simulink model "two_chamber_membrane"  (R2025a)
settings: Solver=VariableStepAuto  StartTime=0.0  StopTime=1000000  RelTol=1e-3  AbsTol=1e-3
libraries: nesl_utility x1
settings Model: Creator=degoede  LastModifiedBy=degoede
settings SolverCC: AutoScaleAbsTol=off
settings SimscapeCC: SimscapeLogType=all  SimscapeLogSimulationStatistics=on  SimscapeLogOpenViewer=on

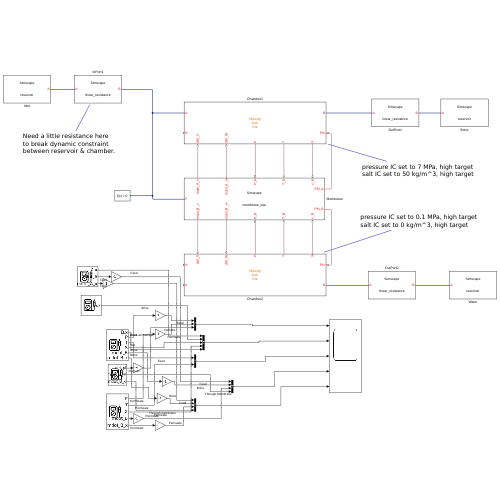
[thumbnail: Simulink's stored preview of the top-level diagram]
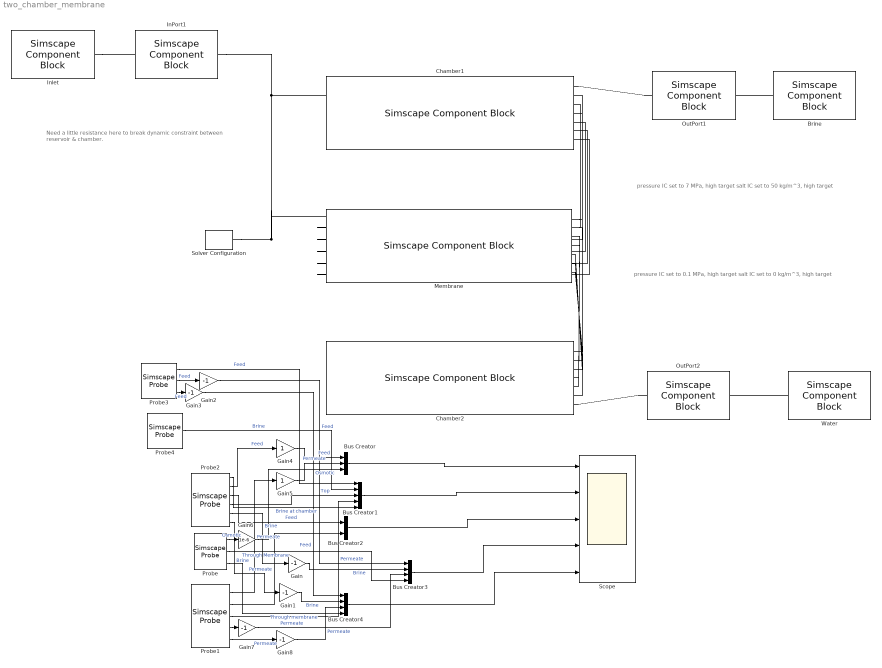
== system two_chamber_membrane ==
  note: pressure IC set to 7 MPa, high target
      | salt IC set to 50 kg/m^3, high target
  note: Need a little resistance here
      | to break dynamic constraint
      | between reservoir & chamber.
  note: pressure IC set to 0.1 MPa, high target
      | salt IC set to 0 kg/m^3, high target
  Brine : SimscapeComponentBlock  SourceFile=customization.solution.elements.reservoir  ComponentPath=customization.solution.elements.reservoir  ComponentVariants="[\"customization.solution.elements.reservoir\"]"  ComponentVariantNames="[\"reservoir\"]"  ClassName=reservoir  SchemaVersion=1  pressure_spec=foundation.enum.pressure_spec.atmospheric  reservoir_pressure=0.101325 MPa  reservoir_temperature=293.15 K  reservoir_concentration=50 kg/m^3  area=1 cm^2
      settings: CopyFcn=simscape.sscblock.internal.componentBlockCallback(gcbh,'COPY')  PreCopyFcn=simscape.sscblock.internal.componentBlockCallback(gcbh,'PRECOPY')  PreDeleteFcn=simscape.sscblock.internal.componentBlockCallback(gcbh,'PREDELETE')  InternalSimscapePortConfiguration="{\"Bottom\":[],\"Left\":[{\"id\":\"A\",\"label\":\"A\",\"type\":\"customization.solution.solution\"}],\"Right\":[],\"Top\":[]}"
      mask Type: Reservoir (SS)
  Bus Creator : BusCreator  Inputs=3
  Bus Creator1 : BusCreator  Inputs=5
  Bus Creator2 : BusCreator  Inputs=2
  Bus Creator3 : BusCreator  Inputs=4
  Bus Creator4 : BusCreator  Inputs=4
  Chamber1 : SimscapeComponentBlock  SourceFile=customization.solution.elements.constant_volume_chamber  ComponentPath=customization.solution.elements.constant_volume_chamber  ComponentVariants="[\"customization.solution.elements.constant_volume_chamber\"]"  ComponentVariantNames="[\"constant_volume_chamber\"]"  ClassName=constant_volume_chamber  SchemaVersion=1  volume=0.001 m^3  num_ports=foundation.enum.num_ports.two  area_A=1 cm^2  area_B=1 cm^2  area_C=0.01 m^2  area_D=0.01 m^2  m_measure=false  p_measure=true  t_measure=true  x_measure=true  p_I_specify=on  p_I_priority=High  p_I=7 MPa  p_I_nominal_specify=off  p_I_nominal_value=1  p_I_nominal_unit=MPa  T_I_specify=off  T_I_priority=High  T_I=293.15 K  T_I_nominal_specify=off  T_I_nominal_value=1  T_I_nominal_unit=K  u_I_specify=off  u_I_priority=None  u_I=83.906 kJ/kg  u_I_nominal_specify=off  u_I_nominal_value=1  u_I_nominal_unit=kJ/kg  rho_I_specify=off  rho_I_priority=None  rho_I=998.21 kg/m^3  rho_I_nominal_specify=off  rho_I_nominal_value=1  rho_I_nominal_unit=kg/m^3  x_I_specify=on  x_I_priority=High  x_I=50 kg/m^3  x_I_nominal_specify=off  x_I_nominal_value=1  x_I_nominal_unit=kg/m^3
      settings: CopyFcn=simscape.sscblock.internal.componentBlockCallback(gcbh,'COPY')  PreCopyFcn=simscape.sscblock.internal.componentBlockCallback(gcbh,'PRECOPY')  PreDeleteFcn=simscape.sscblock.internal.componentBlockCallback(gcbh,'PREDELETE')  InternalSimscapePortConfiguration="{\"Bottom\":[{\"id\":\"dM_X\",\"label\":\"dM_X\",\"type\":\"input\"},{\"id\":\"dM_W\",\"label\":\"dM_W\",\"type\":\"input\"},{\"id\":\"P\",\"label\":\"P\",\"type\":\"output\"},{\"id\":\"T\",\"label\":\"T\",\"type\":\"output\"},{\"id\":\"X\",\"label\":\"X\",\"type\":\"output\"}],\"Left\":[{\"id\":\"A\",\"label\":\"A\",\"type\":\"customization.solution.solution\"},{\"id\":\"H\",\"label\":\"H\",\"type\":\"foundation.thermal.thermal\"}],\"Right\":[{\"id\":\"B\",\"label\":\"B\",\"type\":\"customization.solution.solution\"},{\"id\":\"Phi\",\"label\":\"Phi\",\"type\":\"input\"}],\"Top\":[]}"
      mask Type: Constant Volume Chamber (SS)
  Chamber2 : SimscapeComponentBlock  SourceFile=customization.solution.elements.constant_volume_chamber  ComponentPath=customization.solution.elements.constant_volume_chamber  ComponentVariants="[\"customization.solution.elements.constant_volume_chamber\"]"  ComponentVariantNames="[\"constant_volume_chamber\"]"  ClassName=constant_volume_chamber  SchemaVersion=1  volume=0.001 m^3  num_ports=foundation.enum.num_ports.two  area_A=1 cm^2  area_B=1 cm^2  area_C=0.01 m^2  area_D=0.01 m^2  m_measure=false  p_measure=true  t_measure=true  x_measure=true  p_I_specify=on  p_I_priority=High  p_I=0.1 MPa  p_I_nominal_specify=off  p_I_nominal_value=1  p_I_nominal_unit=MPa  T_I_specify=off  T_I_priority=High  T_I=293.15 K  T_I_nominal_specify=off  T_I_nominal_value=1  T_I_nominal_unit=K  u_I_specify=off  u_I_priority=None  u_I=83.906 kJ/kg  u_I_nominal_specify=off  u_I_nominal_value=1  u_I_nominal_unit=kJ/kg  rho_I_specify=off  rho_I_priority=None  rho_I=998.21 kg/m^3  rho_I_nominal_specify=off  rho_I_nominal_value=1  rho_I_nominal_unit=kg/m^3  x_I_specify=on  x_I_priority=High  x_I=0 kg/m^3  x_I_nominal_specify=off  x_I_nominal_value=1  x_I_nominal_unit=kg/m^3
      settings: CopyFcn=simscape.sscblock.internal.componentBlockCallback(gcbh,'COPY')  PreCopyFcn=simscape.sscblock.internal.componentBlockCallback(gcbh,'PRECOPY')  PreDeleteFcn=simscape.sscblock.internal.componentBlockCallback(gcbh,'PREDELETE')  InternalSimscapePortConfiguration="{\"Bottom\":[{\"id\":\"dM_X\",\"label\":\"dM_X\",\"type\":\"input\"},{\"id\":\"dM_W\",\"label\":\"dM_W\",\"type\":\"input\"},{\"id\":\"P\",\"label\":\"P\",\"type\":\"output\"},{\"id\":\"T\",\"label\":\"T\",\"type\":\"output\"},{\"id\":\"X\",\"label\":\"X\",\"type\":\"output\"}],\"Left\":[{\"id\":\"A\",\"label\":\"A\",\"type\":\"customization.solution.solution\"},{\"id\":\"H\",\"label\":\"H\",\"type\":\"foundation.thermal.thermal\"}],\"Right\":[{\"id\":\"B\",\"label\":\"B\",\"type\":\"customization.solution.solution\"},{\"id\":\"Phi\",\"label\":\"Phi\",\"type\":\"input\"}],\"Top\":[]}"
      mask Type: Constant Volume Chamber (SS)
  Gain{,1..3,7..8} (6 alike) : Gain  Gain=-1
  Gain4 : Gain
  Gain5 : Gain
  Gain6 : Gain  Gain=1e-6
  InPort1 : SimscapeComponentBlock  SourceFile=customization.solution.elements.linear_resistance  ComponentPath=customization.solution.elements.linear_resistance  ComponentVariants="[\"customization.solution.elements.linear_resistance\"]"  ComponentVariantNames="[\"linear_resistance\"]"  ClassName=linear_resistance  SchemaVersion=1  R=64.23e3 Pa*s/m^3  area=1 cm^2
      settings: CopyFcn=simscape.sscblock.internal.componentBlockCallback(gcbh,'COPY')  PreCopyFcn=simscape.sscblock.internal.componentBlockCallback(gcbh,'PRECOPY')  PreDeleteFcn=simscape.sscblock.internal.componentBlockCallback(gcbh,'PREDELETE')  InternalSimscapePortConfiguration="{\"Bottom\":[],\"Left\":[{\"id\":\"A\",\"label\":\"A\",\"type\":\"customization.solution.solution\"}],\"Right\":[{\"id\":\"B\",\"label\":\"B\",\"type\":\"customization.solution.solution\"}],\"Top\":[]}"
      mask Type: Linear Resistance (SS)
  Inlet : SimscapeComponentBlock  SourceFile=customization.solution.elements.reservoir  ComponentPath=customization.solution.elements.reservoir  ComponentVariants="[\"customization.solution.elements.reservoir\"]"  ComponentVariantNames="[\"reservoir\"]"  ClassName=reservoir  SchemaVersion=1  pressure_spec=foundation.enum.pressure_spec.specified  reservoir_pressure=7 MPa  reservoir_temperature=293.15 K  reservoir_concentration=50 kg/m^3  area=1 cm^2
      settings: CopyFcn=simscape.sscblock.internal.componentBlockCallback(gcbh,'COPY')  PreCopyFcn=simscape.sscblock.internal.componentBlockCallback(gcbh,'PRECOPY')  PreDeleteFcn=simscape.sscblock.internal.componentBlockCallback(gcbh,'PREDELETE')  InternalSimscapePortConfiguration="{\"Bottom\":[],\"Left\":[{\"id\":\"A\",\"label\":\"A\",\"type\":\"customization.solution.solution\"}],\"Right\":[],\"Top\":[]}"
      mask Type: Reservoir (SS)
  Membrane : SimscapeComponentBlock  SourceFile=customization.solution.elements.membrane_eqs  ComponentPath=customization.solution.elements.membrane_eqs  ComponentVariants="[\"customization.solution.elements.membrane_eqs\"]"  ComponentVariantNames="[\"membrane_eqs\"]"  ClassName=membrane_eqs  SchemaVersion=1  A_w=2.57e-12 m^3/(N*s)  B_s=2.30e-8 m/s  A_m=35 m^2
      settings: CopyFcn=simscape.sscblock.internal.componentBlockCallback(gcbh,'COPY')  PreCopyFcn=simscape.sscblock.internal.componentBlockCallback(gcbh,'PRECOPY')  PreDeleteFcn=simscape.sscblock.internal.componentBlockCallback(gcbh,'PREDELETE')  InternalSimscapePortConfiguration="{\"Bottom\":[{\"id\":\"mdot_B_x\",\"label\":\"mdot_B_x\",\"type\":\"output\"},{\"id\":\"mdot_B_w\",\"label\":\"mdot_B_w\",\"type\":\"output\"},{\"id\":\"P_B\",\"label\":\"P_B\",\"type\":\"input\"},{\"id\":\"T_B\",\"label\":\"T_B\",\"type\":\"input\"},{\"id\":\"x_B\",\"label\":\"x_B\",\"type\":\"input\"}],\"Left\":[{\"id\":\"F\",\"label\":\"F\",\"type\":\"customization.solution.solution\"}],\"Right\":[{\"id\":\"Phi_A\",\"label\":\"Phi_A\",\"type\":\"output\"},{\"id\":\"Phi_B\",\"label\":\"Phi_B\",\"type\":\"output\"}],\"Top\":[{\"id\":\"mdot_A_x\",\"label\":\"mdot_A_x\",\"type\":\"output\"},{\"id\":\"mdot_A_w\",\"label\":\"mdot_A_w\",\"type\":\"output\"},{\"id\":\"P_A\",\"label\":\"P_A\",\"type\":\"input\"},{\"id\":\"T_A\",\"label\":\"T_A\",\"type\":\"input\"},{\"id\":\"x_A\",\"label\":\"x_A\",\"type\":\"input\"}]}"
      mask Type: Membrane EQs
  OutPort1 : SimscapeComponentBlock  SourceFile=customization.solution.elements.linear_resistance  ComponentPath=customization.solution.elements.linear_resistance  ComponentVariants="[\"customization.solution.elements.linear_resistance\"]"  ComponentVariantNames="[\"linear_resistance\"]"  ClassName=linear_resistance  SchemaVersion=1  R=64.23e6 Pa*s/m^3  area=1 cm^2
      settings: CopyFcn=simscape.sscblock.internal.componentBlockCallback(gcbh,'COPY')  PreCopyFcn=simscape.sscblock.internal.componentBlockCallback(gcbh,'PRECOPY')  PreDeleteFcn=simscape.sscblock.internal.componentBlockCallback(gcbh,'PREDELETE')  InternalSimscapePortConfiguration="{\"Bottom\":[],\"Left\":[{\"id\":\"A\",\"label\":\"A\",\"type\":\"customization.solution.solution\"}],\"Right\":[{\"id\":\"B\",\"label\":\"B\",\"type\":\"customization.solution.solution\"}],\"Top\":[]}"
      mask Type: Linear Resistance (SS)
  OutPort2 : SimscapeComponentBlock  SourceFile=customization.solution.elements.linear_resistance  ComponentPath=customization.solution.elements.linear_resistance  ComponentVariants="[\"customization.solution.elements.linear_resistance\"]"  ComponentVariantNames="[\"linear_resistance\"]"  ClassName=linear_resistance  SchemaVersion=1  R=64.23e3 Pa*s/m^3  area=1 cm^2
      settings: CopyFcn=simscape.sscblock.internal.componentBlockCallback(gcbh,'COPY')  PreCopyFcn=simscape.sscblock.internal.componentBlockCallback(gcbh,'PRECOPY')  PreDeleteFcn=simscape.sscblock.internal.componentBlockCallback(gcbh,'PREDELETE')  InternalSimscapePortConfiguration="{\"Bottom\":[],\"Left\":[{\"id\":\"A\",\"label\":\"A\",\"type\":\"customization.solution.solution\"}],\"Right\":[{\"id\":\"B\",\"label\":\"B\",\"type\":\"customization.solution.solution\"}],\"Top\":[]}"
      mask Type: Linear Resistance (SS)
  Probe : SimscapeProbe  BoundBlock=1  Variables="{\"del_pi\":{\"Probing\":\"ON\"},\"mdot_B_w\":{\"Probing\":\"ON\"},\"mdot_B_x\":{\"Probing\":\"ON\"},\"rho\":{\"Probing\":\"OFF\"}}"
  Probe1 : SimscapeProbe  BoundBlock=3  Variables="{\"M\":{\"Probing\":\"OFF\"},\"P\":{\"Probing\":\"ON\"},\"T\":{\"Probing\":\"ON\"},\"X\":{\"Probing\":\"ON\"},\"mdot_B\":{\"Probing\":\"ON\"},\"mdot_B_x\":{\"Probing\":\"ON\"}}"
  Probe2 : SimscapeProbe  BoundBlock=2  Variables="{\"B.x\":{\"Probing\":\"ON\"},\"M\":{\"Probing\":\"OFF\"},\"P\":{\"Probing\":\"ON\"},\"T\":{\"Probing\":\"ON\"},\"X\":{\"Probing\":\"ON\"},\"mdot_B\":{\"Probing\":\"ON\"},\"mdot_B_x\":{\"Probing\":\"ON\"}}"
  Probe3 : SimscapeProbe  BoundBlock=7  Variables="{\"A.x\":{\"Probing\":\"ON\"},\"mdot_A\":{\"Probing\":\"ON\"},\"mdot_A_x\":{\"Probing\":\"ON\"}}"
  Probe4 : SimscapeProbe  BoundBlock=5  Variables="{\"A.x\":{\"Probing\":\"ON\"}}"
  Scope : Scope  NumInputPorts=5
      settings: ActiveDisplayString=5  ActiveDisplayYMinimum=-6.2473479121849467E-6  ActiveDisplayYMaximum=5.6226203345922816E-5  YLabel=Solute Flow [kg/s]
  Solver Configuration : nesl_utility/Solver Configuration  PhysicalDomain=network_engine_domain  SubClassName=solver  LeftPortType=input  RightPortType=generic  Tones=[]  Harmonics=[]  SimulateNoise=off  Profile=off  UseLocalSampling=off  EnableSwitchedLinearOptims=on  FrequencyDomain=off  UseCCode=off  RelTol=0.001  AbsTol=0.001  MinStep=1e-09  ToWorkspace=off  RevertToSquareIcSolve=off  NumHomotopyIterations=100  PhasorMode=off  PhasorModeNumHarmonics=1  ConsistencySolver=NEWTON_XTOL_AFTER_FTOL  IndexReductionMethod=DerivativeReplacement  DoDC=off  ResidualTolerance=1e-09  ConsistencyTolSource=GLOBAL  ConsistencyAbsTol=0.001  ConsistencyRelTol=0.001  ConsistencyTolFactor=0.001  UseLocalSolver=off  LocalSolverChoice=NE_BACKWARD_EULER_ADVANCER  ResolveIndetEquations=on  FunctionEvalNumThread=1  LocalSolverSampleTime=0.001  DoFixedCost=off  MaxNonlinIter=3  MaxModeIter=2  ComputeImpulses=off  ImpulseIterations=2  LinearAlgebra=auto  LinearAlgebraNumThread=0  EquationFormulation=NE_TIME_EF  DelaysMemoryBudget=1024  AutomaticFiltering=off  FilteringTimeConstant=0.001  PartitionStorageMethod=AS_NEEDED  PartitionMemoryBudget=1024  PartitionMethod=ROBUST  MultibodyUseLocalSolver=off  MultibodyLocalSolverChoice=ODE1  MultibodyLocalSolverSampleTime=0.001
  Water : SimscapeComponentBlock  SourceFile=customization.solution.elements.reservoir  ComponentPath=customization.solution.elements.reservoir  ComponentVariants="[\"customization.solution.elements.reservoir\"]"  ComponentVariantNames="[\"reservoir\"]"  ClassName=reservoir  SchemaVersion=1  pressure_spec=foundation.enum.pressure_spec.atmospheric  reservoir_pressure=0.101325 MPa  reservoir_temperature=293.15 K  reservoir_concentration=0 kg/m^3  area=1 cm^2
      settings: CopyFcn=simscape.sscblock.internal.componentBlockCallback(gcbh,'COPY')  PreCopyFcn=simscape.sscblock.internal.componentBlockCallback(gcbh,'PRECOPY')  PreDeleteFcn=simscape.sscblock.internal.componentBlockCallback(gcbh,'PREDELETE')  InternalSimscapePortConfiguration="{\"Bottom\":[],\"Left\":[{\"id\":\"A\",\"label\":\"A\",\"type\":\"customization.solution.solution\"}],\"Right\":[],\"Top\":[]}"
      mask Type: Reservoir (SS)
  wires:
  Gain4/1 -> Bus Creator/1  "Feed"
  Gain5/1 -> Bus Creator/2  "Permeate"
  Gain6/1 -> Bus Creator/3  "Osmotic"
  Probe2/4 -> Bus Creator1/3  "Top"
  Probe1/3 -> Bus Creator1/4  "Permeate"
  Probe3/1 -> Bus Creator1/1  "Feed"
  Probe4/1 -> Bus Creator1/2  "Brine"
  Probe2/3 -> Bus Creator2/1  "Feed"
  Probe1/2 -> Bus Creator2/2  "Permeate"
  Gain/1 -> Bus Creator3/2  "Brine"
  Gain7/1 -> Bus Creator3/3  "Permeate"
  Gain2/1 -> Bus Creator3/1  "Feed"
  Gain1/1 -> Bus Creator4/2  "Brine"
  Gain8/1 -> Bus Creator4/3  "Permeate"
  Gain3/1 -> Bus Creator4/1  "Feed"
  Probe/2 -> Bus Creator3/4  "Through Membrane"
  Probe/3 -> Bus Creator4/4  "Through membrane"
  Bus Creator/1 -> Scope/1
  Bus Creator1/1 -> Scope/2
  Bus Creator2/1 -> Scope/3
  Bus Creator3/1 -> Scope/4
  Bus Creator4/1 -> Scope/5
  Probe2/5 -> Gain/1  "Brine"
  Probe2/6 -> Gain1/1  "Brine"
  Probe3/2 -> Gain2/1  "Feed"
  Probe3/3 -> Gain3/1  "Feed"
  Probe2/2 -> Gain4/1  "Feed"
  Probe1/1 -> Gain5/1  "Permeate"
  Probe/1 -> Gain6/1  "Osmotic"
  Probe1/4 -> Gain7/1
  Probe1/5 -> Gain8/1  "Permeate"
  Probe2/1 -> Bus Creator1/5  "Brine at chamber"
  connections:
  Brine/LConn1 -- OutPort1/RConn1
  Solver Configuration/RConn1 -- InPort1/RConn1 -- Chamber1/LConn1 -- Membrane/LConn1
  Inlet/LConn1 -- InPort1/LConn1
  Water/LConn1 -- OutPort2/RConn1
  OutPort2/LConn1 -- Chamber2/RConn1
  OutPort1/LConn1 -- Chamber1/RConn1
  Membrane/LConn2 -- Chamber1/RConn3
  Membrane/LConn3 -- Chamber1/RConn4
  Membrane/LConn4 -- Chamber1/RConn5
  Membrane/LConn5 -- Chamber1/RConn6
  Membrane/LConn6 -- Chamber1/RConn7
  Membrane/RConn3 -- Chamber2/RConn3
  Membrane/RConn4 -- Chamber2/RConn4
  Chamber2/RConn5 -- Membrane/RConn5
  Chamber2/RConn6 -- Membrane/RConn6
  Chamber2/RConn7 -- Membrane/RConn7
  Membrane/RConn2 -- Chamber2/RConn2
  Membrane/RConn1 -- Chamber1/RConn2
